simulink model "routePlanServer"  (R2024a)
settings: Solver=FixedStepDiscrete  StartTime=0.0  StopTime=inf  RelTol=1e-3
model workspace (MAT data in the model file):
  SL_ROS_VariableLengthArrays_MaxSizes.CommonInfo.ArrayTruncateAction = 'EmitWarning'
  SL_ROS_VariableLengthArrays_MaxSizes.MsgTypeMap = containers.Map
  SL_ROS_VariableLengthArrays_MaxSizes.MsgTypeMap.serialization.keys = {'std_msgs/Float64MultiArray', 'std_msgs/Int8MultiArray'}
  SL_ROS_VariableLengthArrays_MaxSizes.MsgTypeMap.serialization.values{1}.PropertyName = 'data'
  SL_ROS_VariableLengthArrays_MaxSizes.MsgTypeMap.serialization.values{1}.DataType = 'double'
  SL_ROS_VariableLengthArrays_MaxSizes.MsgTypeMap.serialization.values{1}.MaxLength = 1500000
  SL_ROS_VariableLengthArrays_MaxSizes.MsgTypeMap.serialization.values{2}.PropertyName = 'data'
  SL_ROS_VariableLengthArrays_MaxSizes.MsgTypeMap.serialization.values{2}.DataType = 'int8'
  SL_ROS_VariableLengthArrays_MaxSizes.MsgTypeMap.serialization.values{2}.MaxLength = 1500000
  SL_ROS_VariableLengthArrays_MaxSizes.MsgTypeMap.serialization.uniformity = 0
  SL_ROS_VariableLengthArrays_MaxSizes.MsgTypeMap.serialization.keyType = 'char'
  SL_ROS_VariableLengthArrays_MaxSizes.MsgTypeMap.serialization.valueType = 'any'
libraries: roshelperlib x4, ros2lib x2, simulink x1
settings Model: Creator=cstabile  LastModifiedBy=cstabile
settings OptimizationCC: EnhancedBackFolding=on  PassReuseOutputArgsAs=Individual arguments  ZeroExternalMemoryAtStartup=off  ZeroInternalMemoryAtStartup=off  MaxStackSize=64  OptimizeBlockOrder=speed  DifferentSizesBufferReuse=on  OptimizationCustomize=off  EfficientTunableParamExpr=on
settings DebuggingCC: ParameterTunabilityLossMsg=error
settings SFSimCC: MATLABDynamicMemAlloc=off
settings RTWCC: Description=Embedded Coder  SystemTargetFile=ert.tlc  HardwareBoard=Robot Operating System 2 (ROS 2)  TLCOptions="-aInlineSetEventsForThisBaseRateFcn=TLC_FALSE -aSuppressMultiTaskScheduler=TLC_FALSE  -aRateBasedStepFcn=0"  TemplateMakefile=ert_default_tmf  Toolchain=Colcon Tools  TargetLang=C++
settings CodeAppCC: ForceParamTrailComments=on  IgnoreCustomStorageClasses=off  OperatorAnnotations=on  SimulinkDataObjDesc=on  SFDataObjDesc=on  InsertBlockDesc=on
settings ERTTargetCC: CodeInterfacePackaging=C++ class  RootIOFormat=Structure reference

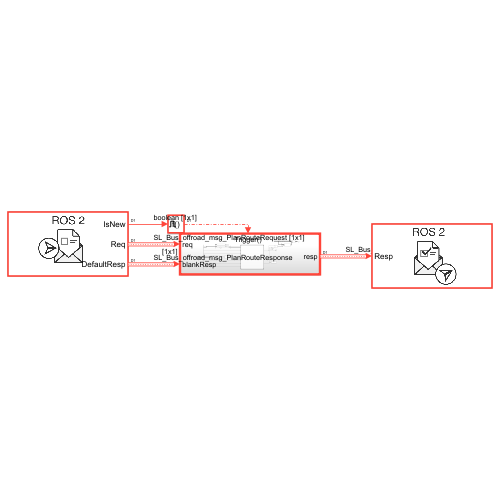
[thumbnail: Simulink's stored preview of the top-level diagram]
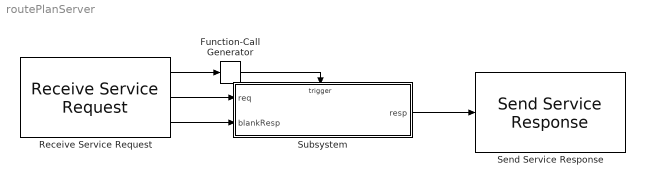
== system routePlanServer ==
  Function-Call Generator : simulink/Ports & Subsystems/Function-Call Generator  sample_time=1  numberOfIterations=1  DisallowWideOutput=off  ShowEnablePort=on
  Receive Service Request : ros2lib/Receive Service Request  service=/planRoute  serviceType=offroad_msg/PlanRoute  SampleTime=-1  ShowDefaultRespOutput=on  BlockId=ServRec_routePlanServer_28  QOSHistory=Keep last  QOSDepth=1  QOSReliability=Reliable  QOSDurability=Volatile  QOSDeadline=Inf  QOSLifespan=Inf  QOSLiveliness=Automatic  QOSLeaseDuration=Inf  QOSAvoidROSNamespaceConventions=off
      settings: LibrarySourceBlock=ros2lib/Receive Request
  Send Service Response : ros2lib/Send Service Response  service=/planRoute  serviceType=offroad_msg/PlanRoute  BlockId=ServRec_routePlanServer_28
      settings: LibrarySourceBlock=ros2lib/Send Response
  Subsystem : Subsystem
  wires:
  Receive Service Request/1 -> Function-Call Generator/1
  Receive Service Request/2 -> Subsystem/1(req)
  Receive Service Request/3 -> Subsystem/2(blankResp)
  Subsystem/1(resp) -> Send Service Response/1
  Function-Call Generator/1 -> Subsystem/Trigger

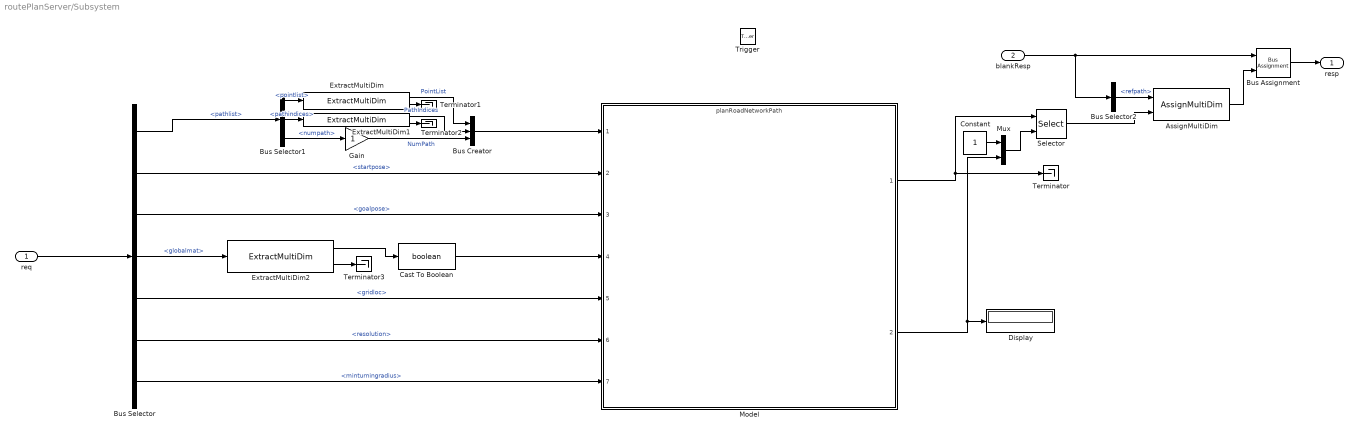
== system routePlanServer/Subsystem ==
  req : Inport
  blankResp : Inport  Port=2
  Trigger : TriggerPort  TriggerType=function-call  VariantControl=(inherit)  OutputDataType=int8  PortDimensions=1
  AssignMultiDim : roshelperlib/AssignMultiDim  SystemSampleTime=-1  VariantActivationTime=update diagram  AllowFlexibleInterface=on  Latency=0  AutoFrameSizeCalculation=off
  Bus Assignment : BusAssignment  AssignedSignals=refpath
  Bus Creator : BusCreator  Inputs=3
  Bus Selector : BusSelector  OutputSignals=pathlist,startpose,goalpose,globalmat,gridloc,resolution,tuneableterrainawareparams.minturningradius
  Bus Selector1 : BusSelector  OutputSignals=pointlist,pathindices,numpath
  Bus Selector2 : BusSelector  OutputSignals=refpath
  Cast To Boolean : DataTypeConversion  OutDataTypeStr=boolean  SaturateOnIntegerOverflow=off  RndMeth=Floor
  Constant : Constant
  Display : Display
  ExtractMultiDim : roshelperlib/ExtractMultiDim  userDataType=double  dims=[1e5 2]  isVarsize=off  varsizeDims=[]  returnFixedTF=off
  ExtractMultiDim1 : roshelperlib/ExtractMultiDim  userDataType=double  dims=[1e3 2]  isVarsize=off  varsizeDims=[]  returnFixedTF=off
  ExtractMultiDim2 : roshelperlib/ExtractMultiDim  userDataType=int8  dims=[1201 1201]  isVarsize=off  varsizeDims=[]  returnFixedTF=off
  Gain : Gain
  Model : ModelReference  ModelNameDialog=planRoadNetworkPath.slx  SimulationMode=Normal  ModelReferenceVersion=1.0
  Mux : Mux  Inputs=2
  Selector : Selector  NumberOfDimensions=2  InputPortWidth=3  IndexOptions=Starting and ending indices (port),Select all  Indices=[1 3],1  OutputSizes=1,1
  Terminator{,1..3} (4 alike) : Terminator
  resp : Outport
  wires:
  Model/1 -> Selector/1, Terminator/1
  Model/2 -> Mux/2, Display/1
  req/1 -> Bus Selector/1
  Bus Selector/1 -> Bus Selector1/1  "<pathlist>"
  Bus Selector1/1 -> ExtractMultiDim/1  "<pointlist>"
  ExtractMultiDim/2 -> Terminator1/1
  Bus Selector1/2 -> ExtractMultiDim1/1  "<pathindices>"
  ExtractMultiDim1/2 -> Terminator2/1
  ExtractMultiDim1/1 -> Bus Creator/2  "PathIndices"
  ExtractMultiDim/1 -> Bus Creator/1  "PointList"
  Bus Selector1/3 -> Gain/1  "<numpath>"
  Gain/1 -> Bus Creator/3  "NumPath"
  blankResp/1 -> Bus Assignment/1, Bus Selector2/1
  Bus Selector2/1 -> AssignMultiDim/1  "<refpath>"
  AssignMultiDim/1 -> Bus Assignment/2
  Bus Assignment/1 -> resp/1
  Selector/1 -> AssignMultiDim/2
  Mux/1 -> Selector/2
  Constant/1 -> Mux/1
  Bus Creator/1 -> Model/1
  Bus Selector/2 -> Model/2  "<startpose>"
  Bus Selector/3 -> Model/3  "<goalpose>"
  Bus Selector/4 -> ExtractMultiDim2/1  "<globalmat>"
  Bus Selector/5 -> Model/5  "<gridloc>"
  Bus Selector/6 -> Model/6  "<resolution>"
  Bus Selector/7 -> Model/7  "<minturningradius>"
  Cast To Boolean/1 -> Model/4
  ExtractMultiDim2/1 -> Cast To Boolean/1
  ExtractMultiDim2/2 -> Terminator3/1
